simulink library "angle_lib"  (R2021a)
settings: Solver=VariableStepAuto  StartTime=0.0  StopTime=10.0  RelTol=1e-3
settings Model: Creator=tshintai  LastModifiedBy=tshintai

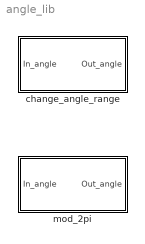
== system angle_lib ==
  change_angle_range : Subsystem
  mod_2pi : Subsystem

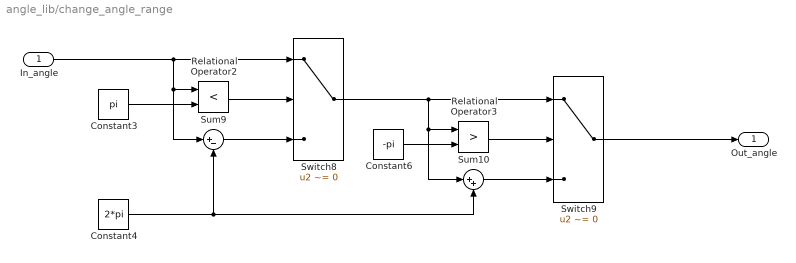
== system angle_lib/change_angle_range ==
  In_angle : Inport
  Constant3 : Constant  Value=pi  OutDataTypeStr=Inherit: Inherit via back propagation
  Constant4 : Constant  Value=2*pi  OutDataTypeStr=Inherit: Inherit via back propagation
  Constant6 : Constant  Value=-pi  OutDataTypeStr=Inherit: Inherit via back propagation
  Relational Operator2 : RelationalOperator  Operator=<  OutDataTypeStr=boolean  RndMeth=Nearest
  Relational Operator3 : RelationalOperator  Operator=>  OutDataTypeStr=boolean  RndMeth=Nearest
  Sum10 : Sum  Inputs=|++
  Sum9 : Sum  Inputs=|+-
  Switch8 : Switch  Criteria=u2 ~= 0
  Switch9 : Switch  Criteria=u2 ~= 0
  Out_angle : Outport
  wires:
  Constant6/1 -> Relational Operator3/2
  Relational Operator2/1 -> Switch8/2
  In_angle/1 -> Relational Operator2/1, Sum9/1, Switch8/1
  Relational Operator3/1 -> Switch9/2
  Constant3/1 -> Relational Operator2/2
  Constant4/1 -> Sum10/2, Sum9/2
  Sum10/1 -> Switch9/3
  Switch8/1 -> Relational Operator3/1, Sum10/1, Switch9/1
  Sum9/1 -> Switch8/3
  Switch9/1 -> Out_angle/1

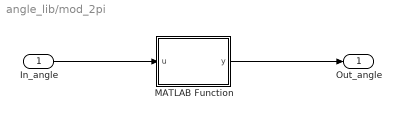
== system angle_lib/mod_2pi ==
  In_angle : Inport
  MATLAB Function : MATLAB Function  TreatAsAtomicUnit=on
  Out_angle : Outport
  wires:
  MATLAB Function/1(y) -> Out_angle/1
  In_angle/1 -> MATLAB Function/1(u)

== matlab function angle_lib/mod_2pi/MATLAB Function ==
  data: u input; y output
function y = fcn(u)

TWO_PI = 2*pi;
input = u;

if (input >= 0)
    while (input > TWO_PI)
        input = input - TWO_PI;
    end
else
    while (input < -TWO_PI)
        input = input + TWO_PI;
    end
end

y = input;

end
